simulink model "model1"  (R2019b)
settings: Solver=VariableStepAuto  StartTime=0.0  StopTime=5  RelTol=1e-3
values from neighbouring files (symbols this model uses):
  K = 1    [zad1.m]
  T = 1    [zad1.m]
undefined symbols (not defined in the file or in its folder): licz1, licz2, mian1, mian2
settings Model: Creator=Szymon  LastModifiedBy=marci

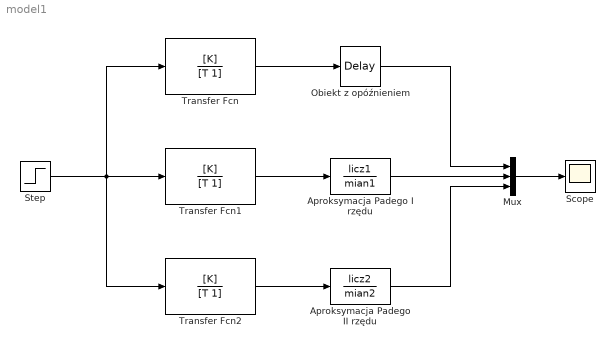
== system model1 ==
  Aproksymacja Padego I rzędu : TransferFcn  Numerator=licz1  Denominator=mian1
  Aproksymacja Padego II rzędu : TransferFcn  Numerator=licz2  Denominator=mian2
  Mux : Mux  Inputs=3
  Obiekt z opóźnieniem : TransportDelay
  Scope : Scope
  Step : Step  Time=0  SampleTime=0
  Transfer Fcn : TransferFcn  Numerator=[K]  Denominator=[T 1]
  Transfer Fcn1 : TransferFcn  Numerator=[K]  Denominator=[T 1]
  Transfer Fcn2 : TransferFcn  Numerator=[K]  Denominator=[T 1]
  wires:
  Step/1 -> Transfer Fcn2/1, Transfer Fcn/1, Transfer Fcn1/1
  Transfer Fcn1/1 -> Aproksymacja Padego I rzędu/1
  Transfer Fcn/1 -> Obiekt z opóźnieniem/1
  Transfer Fcn2/1 -> Aproksymacja Padego II rzędu/1
  Aproksymacja Padego I rzędu/1 -> Mux/2
  Obiekt z opóźnieniem/1 -> Mux/1
  Aproksymacja Padego II rzędu/1 -> Mux/3
  Mux/1 -> Scope/1
